simulink model "final_model_waypoints"  (R2024b)
settings: Solver=FixedStepAuto  StartTime=0.0  StopTime=inf  FixedStep=0.001  RelTol=1e-3
InitFcn:
  | Ts = 0.01;
model workspace (MAT data in the model file):
  SL_ROS_VariableLengthArrays_MaxSizes.CommonInfo.ArrayTruncateAction = 'EmitWarning'
  SL_ROS_VariableLengthArrays_MaxSizes.MsgTypeMap = containers.Map
  SL_ROS_VariableLengthArrays_MaxSizes.MsgTypeMap.serialization.keys = {'sensor_msgs/LaserScan', 'std_msgs/MultiArrayDimension', 'std_msgs/MultiArrayLayout', 'std_msgs/UInt8MultiArray'}
  SL_ROS_VariableLengthArrays_MaxSizes.MsgTypeMap.serialization.values{1}(1).PropertyName = 'intensities'
  SL_ROS_VariableLengthArrays_MaxSizes.MsgTypeMap.serialization.values{1}(1).DataType = 'single'
  SL_ROS_VariableLengthArrays_MaxSizes.MsgTypeMap.serialization.values{1}(1).MaxLength = 360
  SL_ROS_VariableLengthArrays_MaxSizes.MsgTypeMap.serialization.values{1}(2).PropertyName = 'ranges'
  SL_ROS_VariableLengthArrays_MaxSizes.MsgTypeMap.serialization.values{1}(2).DataType = 'single'
  SL_ROS_VariableLengthArrays_MaxSizes.MsgTypeMap.serialization.values{1}(2).MaxLength = 360
  SL_ROS_VariableLengthArrays_MaxSizes.MsgTypeMap.serialization.values{2}.PropertyName = 'label'
  SL_ROS_VariableLengthArrays_MaxSizes.MsgTypeMap.serialization.values{2}.DataType = 'uint8'
  SL_ROS_VariableLengthArrays_MaxSizes.MsgTypeMap.serialization.values{2}.MaxLength = 4
  SL_ROS_VariableLengthArrays_MaxSizes.MsgTypeMap.serialization.values{3}.PropertyName = 'dim'
  SL_ROS_VariableLengthArrays_MaxSizes.MsgTypeMap.serialization.values{3}.DataType = 'std_msgs/MultiArrayDimension'
  SL_ROS_VariableLengthArrays_MaxSizes.MsgTypeMap.serialization.values{3}.MaxLength = 1
  SL_ROS_VariableLengthArrays_MaxSizes.MsgTypeMap.serialization.values{4}.PropertyName = 'data'
  SL_ROS_VariableLengthArrays_MaxSizes.MsgTypeMap.serialization.values{4}.DataType = 'uint8'
  SL_ROS_VariableLengthArrays_MaxSizes.MsgTypeMap.serialization.values{4}.MaxLength = 16
  SL_ROS_VariableLengthArrays_MaxSizes.MsgTypeMap.serialization.uniformity = 0
  SL_ROS_VariableLengthArrays_MaxSizes.MsgTypeMap.serialization.keyType = 'char'
  SL_ROS_VariableLengthArrays_MaxSizes.MsgTypeMap.serialization.valueType = 'any'
values from neighbouring files (symbols this model uses):
  scan = lidarScan(ranges, angles)    [VFHSystem.m]    (also in VFH_ROS.m)
libraries: ros2lib x5, svdutilitieslib x3, sharedtransform x1
settings Model: Creator=01149  LastModifiedBy=01149
settings OptimizationCC: DefaultParameterBehavior=Inlined  EnhancedBackFolding=on  PassReuseOutputArgsAs=Individual arguments  ZeroExternalMemoryAtStartup=off  ZeroInternalMemoryAtStartup=off  MaxStackSize=64  OptimizeBlockOrder=speed  DifferentSizesBufferReuse=on  OptimizationCustomize=off  EfficientTunableParamExpr=on
settings DebuggingCC: ParameterTunabilityLossMsg=error
settings HardwareCC: ProdBitPerLong=64  ProdLargestAtomicInteger=LongLong  ProdLargestAtomicFloat=Double  ProdLongLongMode=on  ProdHWDeviceType=ARM Compatible->ARM Cortex-A (64-bit)
settings RTWCC: Description=Embedded Coder  SystemTargetFile=ert.tlc  HardwareBoard=Robot Operating System 2 (ROS 2)  TLCOptions="-aInlineSetEventsForThisBaseRateFcn=TLC_FALSE -aSuppressMultiTaskScheduler=TLC_FALSE  -aRateBasedStepFcn=0"  TemplateMakefile=ert_default_tmf  Toolchain=Colcon Tools  TargetLang=C++
settings CodeAppCC: ForceParamTrailComments=on  IgnoreCustomStorageClasses=off  OperatorAnnotations=on  SimulinkDataObjDesc=on  SFDataObjDesc=on  InsertBlockDesc=on
settings ERTTargetCC: CodeInterfacePackaging=C++ class  RootIOFormat=Structure reference

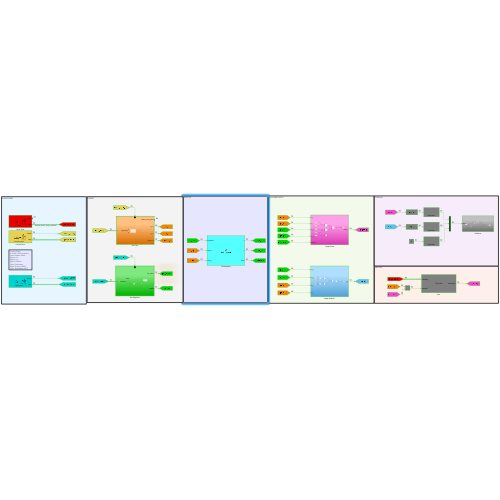
[thumbnail: Simulink's stored preview of the top-level diagram]
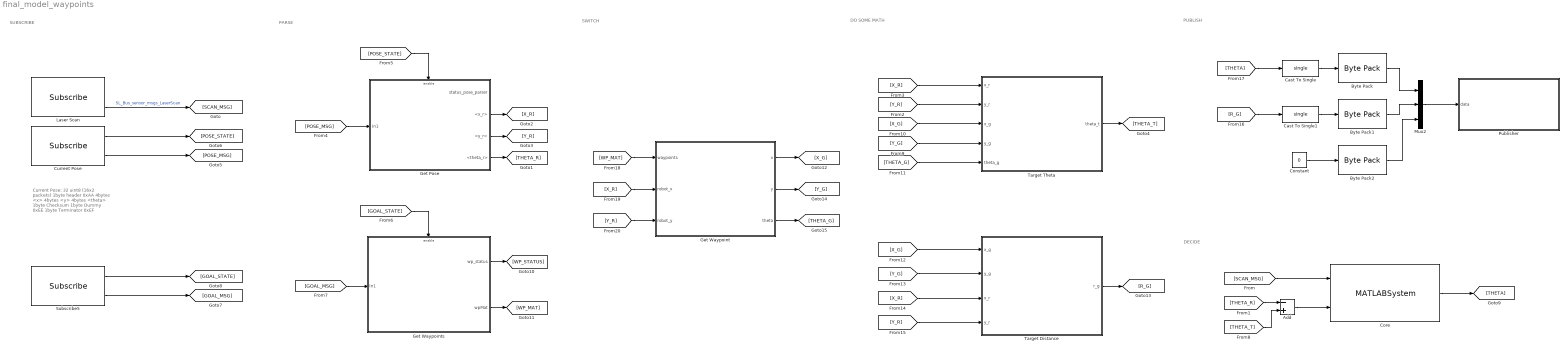
== system final_model_waypoints ==
  note: SWITCH
  note: DECIDE
  note: PUBLISH
  note: DO SOME MATH
  note: PARSE
  note: SUBSCRIBE
  note: Current Pose:
      | 32 uint8 (16x2 packets)
      | 1byte header 0xAA
      | 4bytes <x>
      | 4bytes <y>
      | 4bytes <theta>
      | 1byte Checksum
      | 1byte Dummy 0xEE
      | 1byte Terminator 0xEF
  Add : Sum  Inputs=-+
  Byte Pack : svdutilitieslib/Byte Pack  maskPackedDataType=uint8  datatypes={'single'}  byteAlign=1  blockPlatform=arduinoert
  Byte Pack1 : svdutilitieslib/Byte Pack  maskPackedDataType=uint8  datatypes={'single'}  byteAlign=1  blockPlatform=arduinoert
  Byte Pack2 : svdutilitieslib/Byte Pack  maskPackedDataType=uint8  datatypes={'double'}  byteAlign=1  blockPlatform=arduinoert
  Cast To Single : DataTypeConversion  OutDataTypeStr=single  SaturateOnIntegerOverflow=off  RndMeth=Floor
  Cast To Single1 : DataTypeConversion  OutDataTypeStr=single  SaturateOnIntegerOverflow=off  RndMeth=Floor
  Constant : Constant  Value=0  OutDataTypeStr=double  SampleTime=Ts
  "Core " : MATLABSystem  System=VFH_ROS  DistanceLimits=[ 0.2, 1 ]  RobotRadius=0.3  SafetyDistance=0.2  MinTurningRadius=0.3  SimulateUsing=Code generation
      mask Type: VFH_ROS
      mask Display:
      | disp('VFH_ROS');
      | port_label('input',1,'scanMsg');
      | port_label('input',2,'targetDir');
      | port_label('output',1,'steeringDir');
  Current Pose : ros2lib/Subscribe  topicSource=Select from ROS network  topic=/current_pose  messageType=std_msgs/UInt8MultiArray  sampleTime=Ts  QOSHistory=Keep last  QOSDepth=1  QOSReliability=Reliable  QOSDurability=Volatile  QOSDeadline=Inf  QOSLifespan=Inf  QOSLiveliness=Automatic  QOSLeaseDuration=Inf  QOSAvoidROSNamespaceConventions=off
  "Get Pose " : Subsystem
  Get Waypoint : MATLAB Function  TreatAsAtomicUnit=on
  Get Waypoints : Subsystem
  Laser Scan : ros2lib/Subscribe  topicSource=Specify your own  topic=/scan  messageType=sensor_msgs/LaserScan  sampleTime=Ts  QOSHistory=Keep last  QOSDepth=5  QOSReliability=Best effort  QOSDurability=Volatile  QOSDeadline=Inf  QOSLifespan=Inf  QOSLiveliness=Automatic  QOSLeaseDuration=Inf  QOSAvoidROSNamespaceConventions=off
  Mux2 : Mux  Inputs=3
  Publisher : Subsystem
  Subscribe5 : ros2lib/Subscribe  topicSource=Specify your own  topic=/goal_pose  messageType=geometry_msgs/PoseStamped  sampleTime=Ts  QOSHistory=Keep last  QOSDepth=1  QOSReliability=Reliable  QOSDurability=Volatile  QOSDeadline=Inf  QOSLifespan=Inf  QOSLiveliness=Automatic  QOSLeaseDuration=Inf  QOSAvoidROSNamespaceConventions=off
  "Target Distance " : Subsystem
  Target Theta : Subsystem
  wires:
  Cast To Single/1 -> Byte Pack/1
  Cast To Single1/1 -> Byte Pack1/1
  Byte Pack/1 -> Mux2/1
  Byte Pack1/1 -> Mux2/2
  Mux2/1 -> Publisher/1(data)
  Constant/1 -> Byte Pack2/1
  Byte Pack2/1 -> Mux2/3
  Add/1 -> "Core "/2
  Laser Scan/2 -> [SCAN_MSG]  "SL_Bus_sensor_msgs_LaserScan"
  [SCAN_MSG] -> "Core "/1
  Target Theta/1(theta_t) -> [THETA_T]
  "Get Pose "/4(<theta_r>) -> [THETA_R]
  Current Pose/2 -> [POSE_MSG]
  [POSE_MSG] -> "Get Pose "/1(In1)
  Current Pose/1 -> [POSE_STATE]
  [POSE_STATE] -> "Get Pose "/Enable
  Subscribe5/2 -> [GOAL_MSG]
  Subscribe5/1 -> [GOAL_STATE]
  [GOAL_STATE] -> Get Waypoints/Enable
  [GOAL_MSG] -> Get Waypoints/1(In1)
  "Get Pose "/3(<y_r>) -> [Y_R]
  "Get Pose "/2(<x_r>) -> [X_R]
  [THETA_R] -> Add/1
  [X_R] -> Target Theta/1(x_r)
  [Y_R] -> Target Theta/2(y_r)
  [X_G] -> Target Theta/3(x_g)
  [Y_G] -> Target Theta/4(y_g)
  [THETA_G] -> Target Theta/5(theta_g)
  [THETA_T] -> Add/2
  [X_G] -> "Target Distance "/1(x_g)
  [Y_G] -> "Target Distance "/2(y_g)
  [X_R] -> "Target Distance "/3(x_r)
  [Y_R] -> "Target Distance "/4(y_r)
  "Target Distance "/1(r_g) -> [R_G]
  [R_G] -> Cast To Single1/1
  "Core "/1 -> [THETA]
  [THETA] -> Cast To Single/1
  Get Waypoints/1(wp_status) -> [WP_STATUS]
  Get Waypoints/2(wpMat) -> [WP_MAT]
  Get Waypoint/1(x) -> [X_G]
  Get Waypoint/2(y) -> [Y_G]
  [WP_MAT] -> Get Waypoint/1(waypoints)
  [X_R] -> Get Waypoint/2(robot_x)
  [Y_R] -> Get Waypoint/3(robot_y)
  Get Waypoint/3(theta) -> [THETA_G]

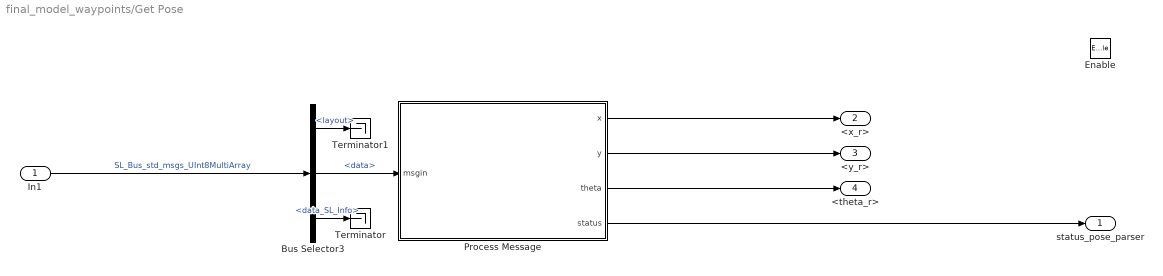
== system final_model_waypoints/Get Pose  ==
  In1 : Inport
  Enable : EnablePort
  Bus Selector3 : BusSelector  OutputSignals=layout,data,data_SL_Info
  Process Message : MATLAB Function  TreatAsAtomicUnit=on
  Terminator : Terminator
  Terminator1 : Terminator
  status_pose_parser : Outport
  <x_r> : Outport  Port=2
  <y_r> : Outport  Port=3
  <theta_r> : Outport  Port=4
  wires:
  In1/1 -> Bus Selector3/1  "SL_Bus_std_msgs_UInt8MultiArray"
  Bus Selector3/2 -> Process Message/1(msgin)  "<data>"
  Process Message/2(y) -> <y_r>/1
  Process Message/4(status) -> status_pose_parser/1
  Process Message/3(theta) -> <theta_r>/1
  Process Message/1(x) -> <x_r>/1
  Bus Selector3/3 -> Terminator/1  "<data_SL_Info>"
  Bus Selector3/1 -> Terminator1/1  "<layout>"

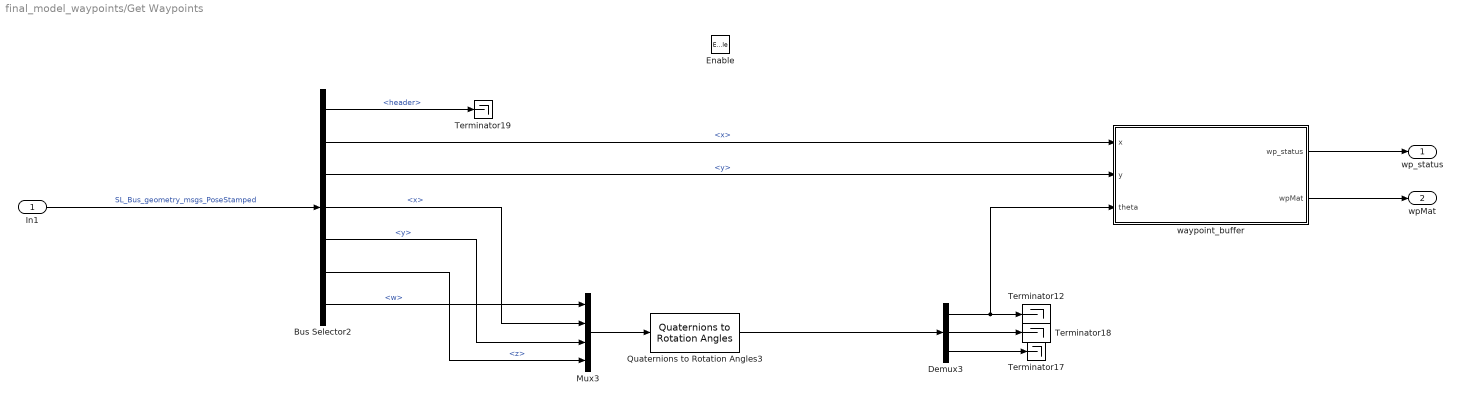
== system final_model_waypoints/Get Waypoints ==
  In1 : Inport
  Enable : EnablePort
  Bus Selector2 : BusSelector  OutputSignals=header,pose.position.x,pose.position.y,pose.orientation.x,pose.orientation.y,pose.orientation.z,pose.orientation.w
  Demux3 : Demux  Outputs=3
  Mux3 : Mux
  Quaternions to Rotation Angles3 : sharedtransform/Quaternions to Rotation Angles  rotationOrder=ZYX  aMode=aMode
  Terminator{12,17..19} (4 alike) : Terminator
  waypoint_buffer : MATLAB Function  TreatAsAtomicUnit=on
  wp_status : Outport
  wpMat : Outport  Port=2
  wires:
  Mux3/1 -> Quaternions to Rotation Angles3/1
  Quaternions to Rotation Angles3/1 -> Demux3/1
  Bus Selector2/7 -> Mux3/1  "<w>"
  Bus Selector2/1 -> Terminator19/1  "<header>"
  Bus Selector2/6 -> Mux3/4  "<z>"
  Bus Selector2/5 -> Mux3/3  "<y>"
  Bus Selector2/2 -> waypoint_buffer/1(x)  "<x>"
  Demux3/3 -> Terminator17/1
  Demux3/1 -> waypoint_buffer/3(theta), Terminator12/1
  Demux3/2 -> Terminator18/1
  Bus Selector2/4 -> Mux3/2  "<x>"
  In1/1 -> Bus Selector2/1  "SL_Bus_geometry_msgs_PoseStamped"
  Bus Selector2/3 -> waypoint_buffer/2(y)  "<y>"
  waypoint_buffer/1(wp_status) -> wp_status/1
  waypoint_buffer/2(wpMat) -> wpMat/1

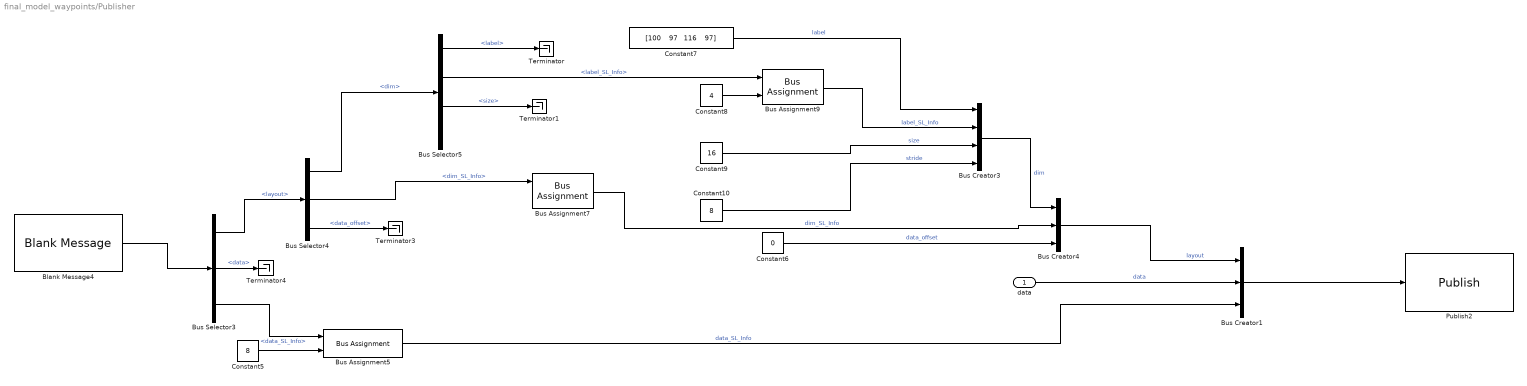
== system final_model_waypoints/Publisher ==
  data : Inport
  Blank Message4 : ros2lib/Blank Message  messageClass=Message  entityType=std_msgs/UInt8MultiArray  messageType=std_msgs/UInt8MultiArray  SampleTime=Ts
  Bus Assignment5 : BusAssignment  AssignedSignals=CurrentLength
  Bus Assignment7 : BusAssignment  AssignedSignals=CurrentLength
  Bus Assignment9 : BusAssignment  AssignedSignals=CurrentLength
  Bus Creator1 : BusCreator  Inputs=3  OutDataTypeStr=Bus: SL_Bus_std_msgs_UInt8MultiArray  NonVirtualBus=on
  Bus Creator3 : BusCreator  Inputs=4  OutDataTypeStr=Bus: SL_Bus_std_msgs_MultiArrayDimension  NonVirtualBus=on
  Bus Creator4 : BusCreator  Inputs=3  OutDataTypeStr=Bus: SL_Bus_std_msgs_MultiArrayLayout  NonVirtualBus=on
  Bus Selector3 : BusSelector  OutputSignals=layout,data,data_SL_Info
  Bus Selector4 : BusSelector  OutputSignals=dim,dim_SL_Info,data_offset
  Bus Selector5 : BusSelector  OutputSignals=label,label_SL_Info,size,stride
  Constant10 : Constant  Value=8  OutDataTypeStr=uint32  SampleTime=Ts
  Constant5 : Constant  Value=8  OutDataTypeStr=uint32  SampleTime=Ts
  Constant6 : Constant  Value=0  OutDataTypeStr=uint32  SampleTime=Ts
  Constant7 : Constant  Value="[100    97   116    97]"  OutDataTypeStr=uint8  SampleTime=Ts
  Constant8 : Constant  Value=4  OutDataTypeStr=uint32  SampleTime=Ts
  Constant9 : Constant  Value=16  OutDataTypeStr=uint32  SampleTime=Ts
  Publish2 : ros2lib/Publish  topicSource=Select from ROS network  topic=/desired_theta  messageType=std_msgs/UInt8MultiArray  QOSHistory=Keep last  QOSDepth=1  QOSReliability=Reliable  QOSDurability=Volatile  QOSDeadline=Inf  QOSLifespan=Inf  QOSLiveliness=Automatic  QOSLeaseDuration=Inf  QOSAvoidROSNamespaceConventions=off
  Terminator{,1,3..4} (4 alike) : Terminator
  wires:
  Constant5/1 -> Bus Assignment5/2
  Bus Assignment9/1 -> Bus Creator3/2  "label_SL_Info"
  Bus Creator3/1 -> Bus Creator4/1  "dim"
  Constant9/1 -> Bus Creator3/3  "size"
  Constant6/1 -> Bus Creator4/3  "data_offset"
  Blank Message4/1 -> Bus Selector3/1
  Bus Creator1/1 -> Publish2/1
  Bus Assignment7/1 -> Bus Creator4/2  "dim_SL_Info"
  Constant7/1 -> Bus Creator3/1  "label"
  Bus Selector4/1 -> Bus Selector5/1  "<dim>"
  Bus Assignment5/1 -> Bus Creator1/3  "data_SL_Info"
  Bus Selector5/2 -> Bus Assignment9/1  "<label_SL_Info>"
  Bus Selector4/2 -> Bus Assignment7/1  "<dim_SL_Info>"
  Bus Selector3/3 -> Bus Assignment5/1  "<data_SL_Info>"
  Constant8/1 -> Bus Assignment9/2
  Constant10/1 -> Bus Creator3/4  "stride"
  Bus Creator4/1 -> Bus Creator1/1  "layout"
  Bus Selector3/1 -> Bus Selector4/1  "<layout>"
  data/1 -> Bus Creator1/2  "data"
  Bus Selector5/1 -> Terminator/1  "<label>"
  Bus Selector5/3 -> Terminator1/1  "<size>"
  Bus Selector4/3 -> Terminator3/1  "<data_offset>"
  Bus Selector3/2 -> Terminator4/1  "<data>"

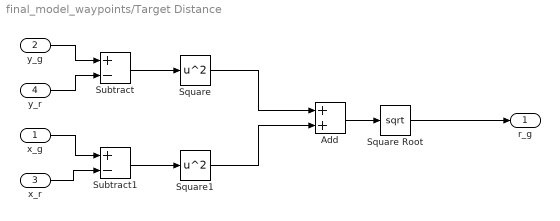
== system final_model_waypoints/Target Distance  ==
  x_g : Inport
  y_g : Inport  Port=2
  x_r : Inport  Port=3
  y_r : Inport  Port=4
  Add : Sum
  Square : Math  Operator=square
  Square Root : Sqrt
  Square1 : Math  Operator=square
  Subtract : Sum  Inputs=+-
  Subtract1 : Sum  Inputs=+-
  r_g : Outport
  wires:
  Add/1 -> Square Root/1
  Square1/1 -> Add/2
  Square/1 -> Add/1
  Square Root/1 -> r_g/1
  y_g/1 -> Subtract/1
  Subtract/1 -> Square/1
  y_r/1 -> Subtract/2
  x_g/1 -> Subtract1/1
  x_r/1 -> Subtract1/2
  Subtract1/1 -> Square1/1

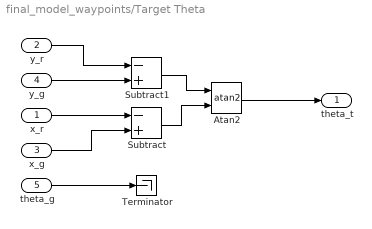
== system final_model_waypoints/Target Theta ==
  x_r : Inport
  y_r : Inport  Port=2
  x_g : Inport  Port=3
  y_g : Inport  Port=4
  theta_g : Inport  Port=5
  Atan2 : Trigonometry  Operator=atan2
  Subtract : Sum  Inputs=-+
  Subtract1 : Sum  Inputs=-+
  Terminator : Terminator
  theta_t : Outport
  wires:
  Subtract1/1 -> Atan2/1
  Atan2/1 -> theta_t/1
  Subtract/1 -> Atan2/2
  theta_g/1 -> Terminator/1
  y_g/1 -> Subtract1/2
  y_r/1 -> Subtract1/1
  x_r/1 -> Subtract/1
  x_g/1 -> Subtract/2

== matlab function final_model_waypoints/Get Waypoint ==
  data: waypoints input; x output; robot_x input; robot_y input; y output; theta output
function [x, y, theta] = nextWaypoint(waypoints, robot_x, robot_y)

    persistent idx numPoints

    if isempty(idx) 
        idx = 1;
        numPoints = size(waypoints, 1);
    end

    x = waypoints(idx, 1);
    y = waypoints(idx, 2);
    theta = waypoints(idx, 3);

    dist = hypot(robot_x - x, robot_y - y);

    if dist <= 1 && idx < numPoints && ~((x+y+theta) == 0)
        idx = idx + 1;
        x = waypoints(idx, 1);
        y = waypoints(idx, 2);
        theta = waypoints(idx, 3);
    end
end

== matlab function final_model_waypoints/Get Waypoints/waypoint_buffer ==
  data: wp_status output uint8; x input; wpMat output; y input; theta input
function [wp_status,wpMat] = waypoint_buffer(x, y, theta)

    persistent buf idx 
    if isempty(buf)
        buf = zeros(10,3);  
        idx = 1;
    end

    if idx <= 10
        buf(idx, :) = [x, y, theta];
        idx = idx + 1;
    end

    if idx > 10
        idx = 1;
        wp_status = uint8(1);
        wpMat = buf;
    else
        wp_status = uint8(0);
        wpMat = zeros(10,3);
    end
end

== matlab function final_model_waypoints/Get Pose /Process Message ==
  data: msgin input uint8; x output; y output; theta output; status output uint8
function [x, y, theta, status] = process_message(msgin)
%#codegen
% process_message searches a 32-element uint8 vector for a valid pose.
%
% A valid packet consists of 16 uint8 elements:
%   Element 1: Header, must equal 0xAA
%   Elements 2-5: Data payload <x> (4 uint8 values)
%   Elements 6-9: Data payload <y> (4 uint8 values)
%   Elements 10-13: Data payload <theta> (4 uint8 values)
%   Element 14: Checksum, XOR(header, data)
%   Element 15: Dummy byte, must equal 0xEE
%   Element 16: Terminator, must equal 0xEF
%
% The function assumes the input chunk is 32 uint8 elements (i.e., 2 times the packet size).
% If a valid packet is found in the current chunk, the payload is updated and returned;
% if not, the last valid payload is returned.
% If two valid packets are found in the same message, the last one is used.
% Ensure that the checksum in the packet and the one between the header and the payload are valid.
% Create a status output with distinct numbers for different states.

% Initialize persistent variables to store the last valid payload
persistent last_x last_y last_theta
if isempty(last_x)
    last_x = 0;
    last_y = 0;
    last_theta = 0;
end

% Initialize status codes
STATUS_NO_PACKET_FOUND = uint8(0);
STATUS_PACKET_FOUND = uint8(1);
STATUS_INVALID_CHECKSUM = uint8(2);

% Initialize output variables
x = last_x;
y = last_y;
theta = last_theta;
status = STATUS_NO_PACKET_FOUND;

% Define packet parameters
PACKET_SIZE = 16;
HEADER = uint8(0xAA);
DUMMY_BYTE = uint8(0xEE);
TERMINATOR = uint8(0xEF);

% Iterate over possible packet start positions in the input vector
for start_idx = 1:(length(msgin) - PACKET_SIZE + 1)
    % Extract potential packet
    packet = msgin(start_idx:start_idx + PACKET_SIZE - 1);

    % Check header, dummy byte, and terminator
    if packet(1) == HEADER && packet(15) == DUMMY_BYTE && packet(16) == TERMINATOR
        % Extract payloads
        x_payload = uint8(packet(2:5));
        y_payload = uint8(packet(6:9));
        theta_payload = uint8(packet(10:13));

        % Convert payloads to single precision floats
        x_candidate = typecast(x_payload, 'single');
        y_candidate = typecast(y_payload, 'single');
        theta_candidate = typecast(theta_payload, 'single');

        % Calculate checksum
        payload = [x_payload, y_payload, theta_payload];

        % Initialize the checksum with the header.
        calculated_checksum = HEADER;
        
        % Iteratively compute the XOR checksum over each payload byte.
        for i = 1:numel(payload)
            calculated_checksum = bitxor(calculated_checksum, payload(i));
        end

        % Validate checksum
        if packet(14) == calculated_checksum
            % Valid packet found; update outputs
            x = double(x_candidate);
            y = double(y_candidate);
            theta = double(theta_candidate);
            status = STATUS_PACKET_FOUND;

            % Update persistent variables
            last_x = x;
            last_y = y;
            theta_converted = mod(theta, 360);
            if theta_converted > 180
                theta_converted = theta_converted - 360; % Shift to [-180, 180]
            end

            last_theta = theta_converted;
        else
            % Invalid checksum
            status = STATUS_INVALID_CHECKSUM;
        end
    end
end
end
